simulink model "CoupledTanks"  (R2023b)
settings: Solver=ode45  StartTime=0.0  StopTime=200  MaxStep=1e-1  RelTol=1e-3  EnableMultiTasking=on
InitFcn:
  | g = 9.81; %gravitational constant
  | 
  | % showVR = 1; %show VR world
  | % h1_init = 0; %initial condition
  | % h2_init = 0; %initial condition
libraries: vrlib x7
CloseFcn:
  | vrclose all;
  | clear figureVR worldVR;
settings Model: Creator=H  LastModifiedBy=pinki
settings SolverCC: AlgebraicLoopSolver=TrustRegion
settings DataIOCC: LimitDataPoints=on  SaveFormat=Array  SignalLoggingSaveFormat=ModelDataLogs  ReturnWorkspaceOutputs=off
settings OptimizationCC: ExpressionDepthLimit=2147483647  InitFltsAndDblsToZero=on  LifeSpan=inf
settings DebuggingCC: SaveWithParameterizedLinksMsg=none  UnderspecifiedInitializationDetection=Classic  MergeDetectMultiDrivingBlocksExec=none  SignalResolutionControl=TryResolveAllWithWarning  SolverPrmCheckMsg=warning  FcnCallInpInsideContextMsg=warning  UnconnectedInputMsg=warning  UnconnectedOutputMsg=warning  UnconnectedLineMsg=warning  StateNameClashWarn=warning  SFUnexpectedBacktrackingDiag=warning  SFNoUnconditionalDefaultTransitionDiag=warning  SFExecutionAtInitializationDiag=none  ArithmeticOperatorsInVariantConditions=warning
settings HardwareCC: ProdBitPerPointer=32  ProdBitPerSizeT=32  ProdBitPerPtrDiffT=32  ProdLargestAtomicFloat=None  ProdIntDivRoundTo=Undefined  ProdEndianess=Unspecified  ProdWordSize=32  ProdHWDeviceType=32-bit Generic
settings ModelReferenceCC: PropagateSignalLabelsOutOfModel=off
settings SFSimCC: SimUseLocalCustomCode=off  CustomCodeUndefinedFunction=UseInterfaceOnly
settings RTWCC: RTWUseLocalCustomCode=off
settings CodeAppCC: StateflowObjectComments=on
settings GRTTargetCC: TargetFcnLib=ansi_tfl_tmw.mat  TargetLangStandard=C89/C90 (ANSI)  CombineOutputUpdateFcns=off  GRTInterface=on
settings ConfigComp: CovMetricSettings=dw  CovSaveCumulativeToWorkspaceVar=on  CovSaveSingleToWorkspaceVar=on  CovExternalEMLEnable=off

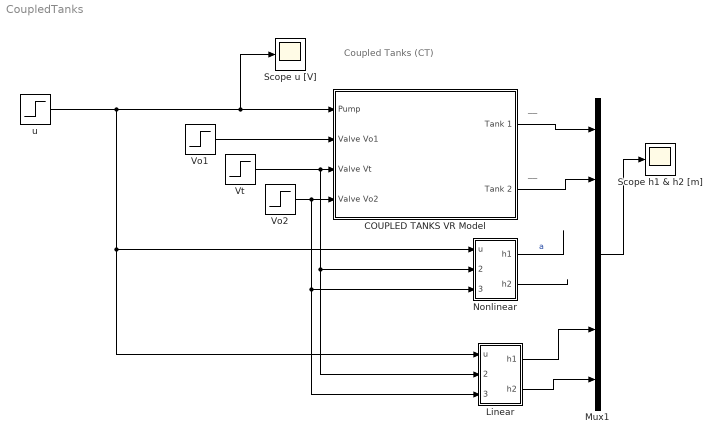
== system CoupledTanks ==
  note: Coupled Tanks (CT)
  note: __
  note: __
  COUPLED TANKS VR Model : Subsystem  mask(Coupled Tanks (CT) in laboratory K26){showVR=off, sfcnParam1=0.2025, sfcnParam2=0.1350}
      mask prompts: showVR "Show VirtualWorld?"; sfcnParam1 "Initial fluid level in the left tank 1   h1(0)  [cm]"; sfcnParam2 "Initial fluid  level in the right tank 2   h2 (0) [cm]"
      mask help:
      | Coupled Tanks (CT) in laboratory K26 - Virtual Reality
      | Real-Time Workshop generated S-function.
      mask Help:
      | Couple Tanks in laboratory K26 - Virtual Reality. <br><br>
      | 
      | 
      | This is a&nbsp;virtual model of the Coupled Tanks apparatus in Laboratory of automatic control
      | theory&nbsp;26 (<a href="http://support.dce.felk.cvut.cz/lab26/" target="_blank">http://support.dce.felk.cvut.cz/lab26/</a>),
      | which consists of a&nbsp;gear-pump, two tanks (left and right), inflow and outflow pipes and transfer (V<sub>t</sub>) and
      | output valves (V<sub>o1</sub>, V<sub>o2</sub>). The&nbsp;left tank is filled with the&nbsp;fluid by the&nbsp;gear-pump
      | controller by the&nbsp;voltage&nbsp;<em>u</em>&nbsp;[V]. The&nbsp;fluid can drain from the&nbsp;left tank through
      | the&nbsp;valve&nbsp;<em>v</em><sub>o1</sub>&nbsp;[%] or can drain to the&nbsp;right tank through the&nbsp;transfer
      | valve&nbsp;<em>v</em><sub>t</sub>&nbsp;[%]. The&nbsp;fluid drains away from the&nbsp;right tank through
      | the&nbsp;valve&nbsp;<em>v</em><sub>o2</sub>&nbsp;[%].<br><br>
      | 
      | The&nbsp;system input are the&nbsp;voltage of the&nbsp;motor of the&nbsp;gear-pump&nbsp;<em>u</em>&nbsp;[V]
      | and the&nbsp;opening of
      | the&nbsp;valves&nbsp;<em>v</em><sub>o1</sub>,&nbsp;<em>v</em><sub>t</sub>,&nbsp;<em>v</em><sub>o2</sub>&nbsp;[%].
      | The&nbsp;system outputs are the&nbsp;levels of the&nbsp;fluid in
      | the&nbsp;tanks&nbsp;<em>h</em><sub>1</sub>,&nbsp;<em>h</em><sub>2</sub>&nbsp;[cm].
      | The&nbsp;dynamics of the&nbsp;gear-pump is neglected. More information can be found on the&nbsp;website
      | <a href="http://support.dce.felk.cvut.cz/lab26/" target="_blank">http://support.dce.felk.cvut.cz/lab26/</a>.<br><br>
      | 
      | 
      | In the mask of the model, it can be set:
      | <ul>
      | <li>Initial fluid level in the left tank</li>
      | <li>Initial fluid level in the right tank.</li>
      | </ul><br><br>
      | 
      | 
      | Copyright: 2008, Jan Kricka, Jirka Roubal, Petr Husek.
      mask Callback showVR:
      | if strcmp('off',get_param(gcb,'showVR'))
      |     vrclose all;
      | else
      |     if exist('figureVR')==0
      |         figureVR = vrfigure;
      |     end
      |     if exist('worldVR')==0
      |         worldVR = vrworld('CoupledTanks_VR.WRL');
      |     end
      | 	if isvalid(figureVR)==0
      |         open(worldVR);
      |         figureVR = vrfigure(worldVR,[650 80 550 350]);
      | 	end
      | end
      mask Display:
      | image(imread('CoupledTanks_Image.jpg'));
      | port_label ('input',1,'u [V]');
      | port_label ('input',2,'Vo1 [-]');
      | port_label ('input',3,'Vt [-]');
      | port_label ('input',4,'Vo2 [-]');
      | port_label ('output',1,'h1 [m]');
      | port_label ('output',2,'h2 [m]');
  Linear : Subsystem
  Mux1 : Mux  Inputs=6
  Nonlinear : Subsystem
  Scope h1 & h2 [m] : Scope
  Scope u [V] : Scope
  Vo1 : Step  Time=0  After=0  SampleTime=0
  Vo2 : Step  Time=0  After=0.3  SampleTime=0
  Vt : Step  Time=0  After=0.2  SampleTime=0
  u : Step  Time=0  After=2.5  SampleTime=0
  wires:
  COUPLED TANKS VR Model/1(Tank 1) -> Mux1/1
  Mux1/1 -> Scope h1 & h2 [m]/1
  Vo1/1 -> COUPLED TANKS VR Model/2(Valve Vo1)
  COUPLED TANKS VR Model/2(Tank 2) -> Mux1/2
  u/1 -> Nonlinear/1(u), Linear/1(u), Scope u [V]/1, COUPLED TANKS VR Model/1(Pump)
  Vt/1 -> Nonlinear/2(V_T), Linear/2(V_T), COUPLED TANKS VR Model/3(Valve Vt)
  Vo2/1 -> Linear/3(V_0), Nonlinear/3(V_0), COUPLED TANKS VR Model/4(Valve Vo2)
  Linear/1(h1) -> Mux1/5
  Linear/2(h2) -> Mux1/6
  Nonlinear/2(h2) -> ?
  Nonlinear/1(h1) -> ?  "a"

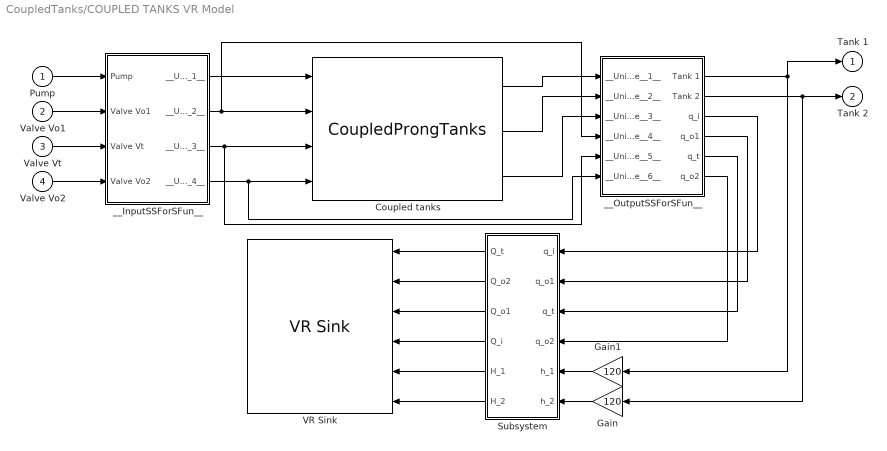
== system CoupledTanks/COUPLED TANKS VR Model ==
  Pump : Inport
  Valve Vo1 : Inport  Port=2
  Valve Vt : Inport  Port=3
  Valve Vo2 : Inport  Port=4
  Coupled tanks : M-S-Function  FunctionName=CoupledProngTanks  Parameters=h10 h20  mask{h10=sfcnParam1, h20=sfcnParam2}
      mask prompts: h10 "h1_init"; h20 "h2_init"
      mask Display:
      | port_label('input',1,'Pump');
      | port_label('input',2,'Valve Vo1');
      | port_label('input',3,'Valve Vt');
      | port_label('input',4,'Valve Vo2');
      | port_label('output',1,'Tank 1');
      | port_label('output',2,'Tank 2');
      | port_label('output',3,'q_i');
  Gain : Gain  Gain=120
  Gain1 : Gain  Gain=120
  Subsystem : Subsystem
  VR Sink : vrlib/VR Sink  InstantiateOnLoad=on  SampleTime=-1  ViewEnable=on  RemoteChange=off  RemoteView=on  FieldsWritten=Valve_t.rotation.4.1.double#Valve_o2.rotation.4.1.double#Valve_o1.rotation.4.1.double#Pump.rotation.4.1.double#water1.scale.3.1.double#water2.scale.3.1.double  WorldFileName=CoupledTanks_VR.WRL  AutoView=off  VideoDimensions=[]  AllowVariableSize=off
  __InputSSForSFun__ : Subsystem
  __OutputSSForSFun__ : Subsystem
  Tank 1 : Outport  OutDataTypeStr=double  PortDimensions=1  SampleTime=[-1 0]
  Tank 2 : Outport  Port=2  OutDataTypeStr=double  PortDimensions=1  SampleTime=[-1 0]
  wires:
  __OutputSSForSFun__/6(q_o2) -> Subsystem/4(q_o2)
  __OutputSSForSFun__/5(q_t) -> Subsystem/3(q_t)
  __OutputSSForSFun__/4(q_o1) -> Subsystem/2(q_o1)
  __OutputSSForSFun__/3(q_i) -> Subsystem/1(q_i)
  Subsystem/2(Q_o2) -> VR Sink/2
  Subsystem/3(Q_o1) -> VR Sink/3
  Subsystem/4(Q_i) -> VR Sink/4
  Subsystem/1(Q_t) -> VR Sink/1
  Subsystem/6(H_2) -> VR Sink/6
  Subsystem/5(H_1) -> VR Sink/5
  __OutputSSForSFun__/2(Tank 2) -> Gain/1, Tank 2/1
  __OutputSSForSFun__/1(Tank 1) -> Tank 1/1, Gain1/1
  __InputSSForSFun__/4(__UniqueOutportName__4__) -> __OutputSSForSFun__/6(__UniqueInportName__6__), Coupled tanks/4
  __InputSSForSFun__/3(__UniqueOutportName__3__) -> __OutputSSForSFun__/5(__UniqueInportName__5__), Coupled tanks/3
  Coupled tanks/2 -> __OutputSSForSFun__/2(__UniqueInportName__2__)
  Coupled tanks/1 -> __OutputSSForSFun__/1(__UniqueInportName__1__)
  __InputSSForSFun__/2(__UniqueOutportName__2__) -> __OutputSSForSFun__/4(__UniqueInportName__4__), Coupled tanks/2
  __InputSSForSFun__/1(__UniqueOutportName__1__) -> Coupled tanks/1
  Valve Vo2/1 -> __InputSSForSFun__/4(Valve Vo2)
  Valve Vt/1 -> __InputSSForSFun__/3(Valve Vt)
  Valve Vo1/1 -> __InputSSForSFun__/2(Valve Vo1)
  Pump/1 -> __InputSSForSFun__/1(Pump)
  Coupled tanks/3 -> __OutputSSForSFun__/3(__UniqueInportName__3__)
  Gain/1 -> Subsystem/6(h_2)
  Gain1/1 -> Subsystem/5(h_1)

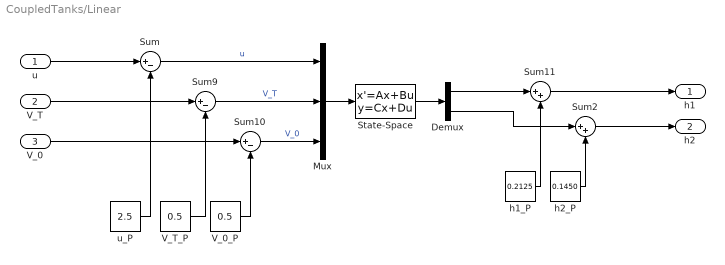
== system CoupledTanks/Linear ==
  u : Inport
  V_T : Inport  Port=2
  V_0 : Inport  Port=3
  Demux : Demux  Outputs=2
  Mux : Mux  Inputs=3
  State-Space : StateSpace  A="[-0.674424,  0.221636; 0.221636, -0.498911]"  B="[0, -0.059842,         0; 0,  0.059842, -0.149728]"  C=[1 0; 0 1]  D=[0 0 0; 0 0 0]  InitialCondition=0
  Sum : Sum  Inputs=|+-
  Sum10 : Sum  Inputs=|+-
  Sum11 : Sum  Inputs=|++
  Sum2 : Sum  Inputs=|++
  Sum9 : Sum  Inputs=|+-
  V_0_P : Constant  Value=0.5
  V_T_P : Constant  Value=0.5
  h1_P : Constant  Value=0.2125
  h2_P : Constant  Value=0.1450
  u_P : Constant  Value=2.5
  h1 : Outport
  h2 : Outport  Port=2
  wires:
  u/1 -> Sum/1
  V_0/1 -> Sum10/1
  State-Space/1 -> Demux/1
  V_T/1 -> Sum9/1
  Sum9/1 -> Mux/2  "V_T"
  Sum/1 -> Mux/1  "u"
  Demux/2 -> Sum2/1
  h1_P/1 -> Sum11/2
  h2_P/1 -> Sum2/2
  Sum11/1 -> h1/1
  V_0_P/1 -> Sum10/2
  V_T_P/1 -> Sum9/2
  Sum10/1 -> Mux/3  "V_0"
  Mux/1 -> State-Space/1
  Demux/1 -> Sum11/1
  u_P/1 -> Sum/2
  Sum2/1 -> h2/1

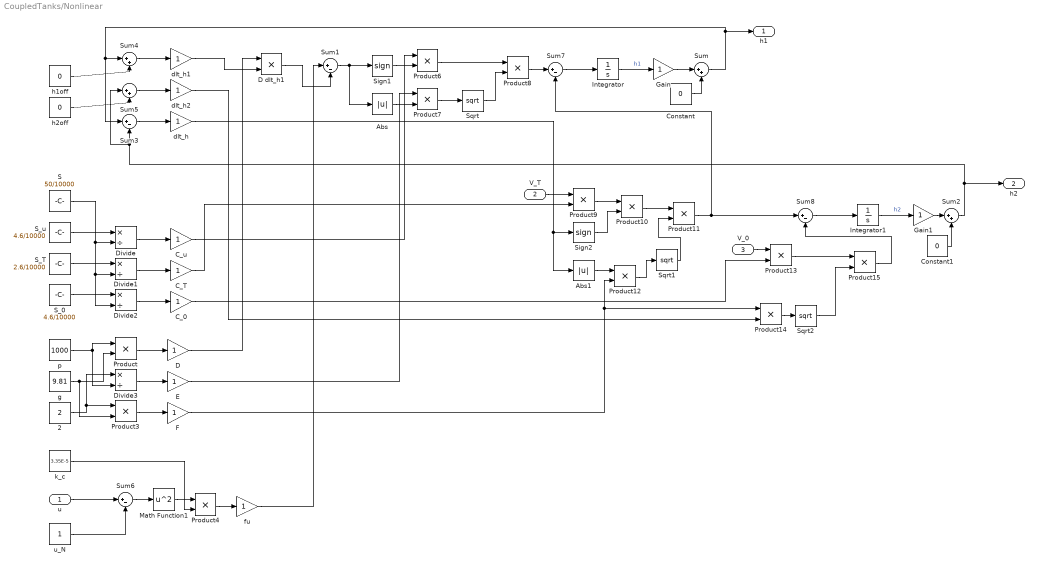
== system CoupledTanks/Nonlinear ==
  u : Inport
  V_T : Inport  Port=2
  V_0 : Inport  Port=3
  2 : Constant  Value=2
  Abs : Abs  SaturateOnIntegerOverflow=off
  Abs1 : Abs  SaturateOnIntegerOverflow=off
  C_0 : Gain
  C_T : Gain
  C_u : Gain
  Constant : Constant  Value=0
  Constant1 : Constant  Value=0
  D : Gain
  D dlt_h1 : Product
  Divide{,1..3} (4 alike) : Product  Inputs=*/
  E : Gain
  F : Gain
  Gain : Gain
  Gain1 : Gain
  Integrator : Integrator  InitialCondition=0.2025
  Integrator1 : Integrator  InitialCondition=0.1350
  Math Function1 : Math  Operator=square
  Product{,3..4,6..15} (13 alike) : Product
  S : Constant  Value=50/10000
  S_0 : Constant  Value=4.6/10000
  S_T : Constant  Value=2.6/10000
  S_u : Constant  Value=4.6/10000
  Sign1 : Signum
  Sign2 : Signum
  Sqrt : Sqrt
  Sqrt1 : Sqrt
  Sqrt2 : Sqrt
  Sum{,2,4..5} (4 alike) : Sum  Inputs=|++
  Sum{1,3,6..8} (5 alike) : Sum  Inputs=|+-
  dlt_h : Gain
  dlt_h1 : Gain
  dlt_h2 : Gain
  fu : Gain
  g : Constant  Value=9.81
  h1off : Constant  Value=0
  h2off : Constant  Value=0
  k_c : Constant  Value=3.35E-5
  p : Constant  Value=1000
  u_N : Constant
  h1 : Outport
  h2 : Outport  Port=2
  wires:
  Integrator1/1 -> Gain1/1  "h2"
  Integrator/1 -> Gain/1  "h1"
  Abs/1 -> Product7/2
  Product14/1 -> Sqrt2/1
  Product15/1 -> Sum8/2
  Product7/1 -> Sqrt/1
  D/1 -> D dlt_h1/1
  Abs1/1 -> Product12/1
  Product6/1 -> Product8/1
  Product10/1 -> Product11/1
  Sum7/1 -> Integrator/1
  Divide1/1 -> C_T/1
  Sqrt1/1 -> Product11/2
  fu/1 -> Sum1/1
  Sign2/1 -> Product10/2
  Sum1/1 -> Abs/1, Sign1/1
  Math Function1/1 -> Product4/1
  Product4/1 -> fu/1
  E/1 -> Product7/1
  V_T/1 -> Product9/1
  Gain1/1 -> Sum2/1
  h1off/1 -> Sum4/2
  Product11/1 -> Sum8/1, Sum7/2
  Product13/1 -> Product15/1
  dlt_h/1 -> Abs1/1, Sign2/1
  Sum6/1 -> Math Function1/1
  u_N/1 -> Sum6/2
  Sum4/1 -> dlt_h1/1
  C_u/1 -> Product6/1
  Sum5/1 -> dlt_h2/1
  C_0/1 -> Product13/2
  Product9/1 -> Product10/1
  Product8/1 -> Sum7/1
  S/1 -> Divide/2, Divide1/2, Divide2/2
  Divide2/1 -> C_0/1
  Sqrt2/1 -> Product15/2
  Sign1/1 -> Product6/2
  Divide/1 -> C_u/1
  Sum8/1 -> Integrator1/1
  dlt_h1/1 -> D dlt_h1/2
  Sqrt/1 -> Product8/2
  Product/1 -> D/1
  D dlt_h1/1 -> Sum1/2
  Sum3/1 -> dlt_h/1
  dlt_h2/1 -> Product14/2
  p/1 -> Divide3/2, Product/1
  C_T/1 -> Product9/2
  S_u/1 -> Divide/1
  2/1 -> Divide3/1, Product3/1
  Product3/1 -> F/1
  g/1 -> Product3/2, Product/2
  h2off/1 -> Sum5/2
  Product12/1 -> Sqrt1/1
  k_c/1 -> Product4/2
  F/1 -> Product14/1, Product12/2
  Divide3/1 -> E/1
  S_0/1 -> Divide2/1
  S_T/1 -> Divide1/1
  V_0/1 -> Product13/1
  u/1 -> Sum6/1
  Sum/1 -> Sum3/1, Sum4/1, h1/1
  Gain/1 -> Sum/1
  Constant/1 -> Sum/2
  Sum2/1 -> Sum5/1, Sum3/2, h2/1
  Constant1/1 -> Sum2/2

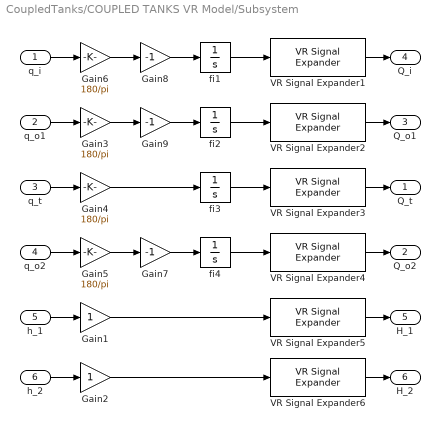
== system CoupledTanks/COUPLED TANKS VR Model/Subsystem ==
  q_i : Inport
  q_o1 : Inport  Port=2
  q_t : Inport  Port=3
  q_o2 : Inport  Port=4
  h_1 : Inport  Port=5
  h_2 : Inport  Port=6
  Gain1 : Gain
  Gain2 : Gain
  Gain{3..6} (4 alike) : Gain  Gain=180/pi
  Gain7 : Gain  Gain=-1
  Gain8 : Gain  Gain=-1
  Gain9 : Gain  Gain=-1
  VR Signal Expander{1..4} (4 alike) : vrlib/VR Signal Expander  outwidth=4  outidx=[4]
  VR Signal Expander5 : vrlib/VR Signal Expander  outwidth=3  outidx=[2]
  VR Signal Expander6 : vrlib/VR Signal Expander  outwidth=3  outidx=[2]
  fi{1..4} (4 alike) : Integrator
  Q_t : Outport
  Q_o2 : Outport  Port=2
  Q_o1 : Outport  Port=3
  Q_i : Outport  Port=4
  H_1 : Outport  Port=5
  H_2 : Outport  Port=6
  wires:
  Gain9/1 -> fi2/1
  Gain8/1 -> fi1/1
  Gain7/1 -> fi4/1
  Gain5/1 -> Gain7/1
  q_o2/1 -> Gain5/1
  VR Signal Expander4/1 -> Q_o2/1
  fi4/1 -> VR Signal Expander4/1
  Gain4/1 -> fi3/1
  Gain6/1 -> Gain8/1
  Gain3/1 -> Gain9/1
  q_t/1 -> Gain4/1
  q_o1/1 -> Gain3/1
  Gain2/1 -> VR Signal Expander6/1
  Gain1/1 -> VR Signal Expander5/1
  VR Signal Expander6/1 -> H_2/1
  VR Signal Expander5/1 -> H_1/1
  VR Signal Expander1/1 -> Q_i/1
  VR Signal Expander2/1 -> Q_o1/1
  VR Signal Expander3/1 -> Q_t/1
  h_2/1 -> Gain2/1
  h_1/1 -> Gain1/1
  q_i/1 -> Gain6/1
  fi2/1 -> VR Signal Expander2/1
  fi3/1 -> VR Signal Expander3/1
  fi1/1 -> VR Signal Expander1/1

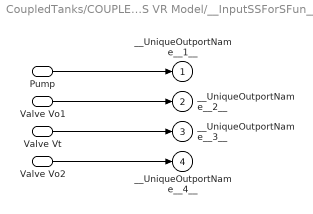
== system CoupledTanks/COUPLED TANKS VR Model/__InputSSForSFun__ ==
  Pump : Inport
  Valve Vo1 : Inport  Port=2
  Valve Vt : Inport  Port=3
  Valve Vo2 : Inport  Port=4
  __UniqueOutportName__1__ : Outport
  __UniqueOutportName__2__ : Outport  Port=2
  __UniqueOutportName__3__ : Outport  Port=3
  __UniqueOutportName__4__ : Outport  Port=4
  wires:
  Valve Vo2/1 -> __UniqueOutportName__4__/1
  Valve Vt/1 -> __UniqueOutportName__3__/1
  Valve Vo1/1 -> __UniqueOutportName__2__/1
  Pump/1 -> __UniqueOutportName__1__/1

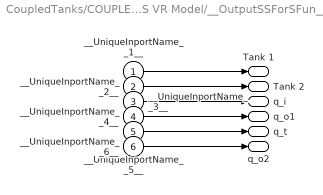
== system CoupledTanks/COUPLED TANKS VR Model/__OutputSSForSFun__ ==
  __UniqueInportName__1__ : Inport
  __UniqueInportName__2__ : Inport  Port=2
  __UniqueInportName__3__ : Inport  Port=3
  __UniqueInportName__4__ : Inport  Port=4
  __UniqueInportName__5__ : Inport  Port=5
  __UniqueInportName__6__ : Inport  Port=6
  Tank 1 : Outport  OutDataTypeStr=double  PortDimensions=1  SampleTime=[-1 0]
  Tank 2 : Outport  Port=2  OutDataTypeStr=double  PortDimensions=1  SampleTime=[-1 0]
  q_i : Outport  Port=3  OutDataTypeStr=double  PortDimensions=1  SampleTime=[0 1]
  q_o1 : Outport  Port=4  OutDataTypeStr=double  PortDimensions=1  SampleTime=[-1 0]
  q_t : Outport  Port=5  OutDataTypeStr=double  PortDimensions=1  SampleTime=[-1 0]
  q_o2 : Outport  Port=6  OutDataTypeStr=double  PortDimensions=1  SampleTime=[-1 0]
  wires:
  __UniqueInportName__6__/1 -> q_o2/1
  __UniqueInportName__5__/1 -> q_t/1
  __UniqueInportName__4__/1 -> q_o1/1
  __UniqueInportName__3__/1 -> q_i/1
  __UniqueInportName__2__/1 -> Tank 2/1
  __UniqueInportName__1__/1 -> Tank 1/1
